simulink model "surgicalControl_Shared_memory_loop_2016a"  (R2016a)
settings: Solver=FixedStepAuto  SolverMode=SingleTasking  StartTime=0.0  StopTime=inf  FixedStep=1/100  RelTol=1e-3
libraries: dspsigops x9, simulink x3, matlabGenericSHM_Block x2
settings Model: Creator=daniel  LastModifiedBy=Bogdan
settings DebuggingCC: SFUnexpectedBacktrackingDiag=error  SFNoUnconditionalDefaultTransitionDiag=error
settings GRTTargetCC: TargetLangStandard=C99 (ISO)  GeneratePreprocessorConditionals=Use local settings
settings ConfigComp: CovMetricSettings=dwe  CovHtmlReporting=off  CovSaveCumulativeToWorkspaceVar=off  CovSaveSingleToWorkspaceVar=off  CovExternalEMLEnable=on

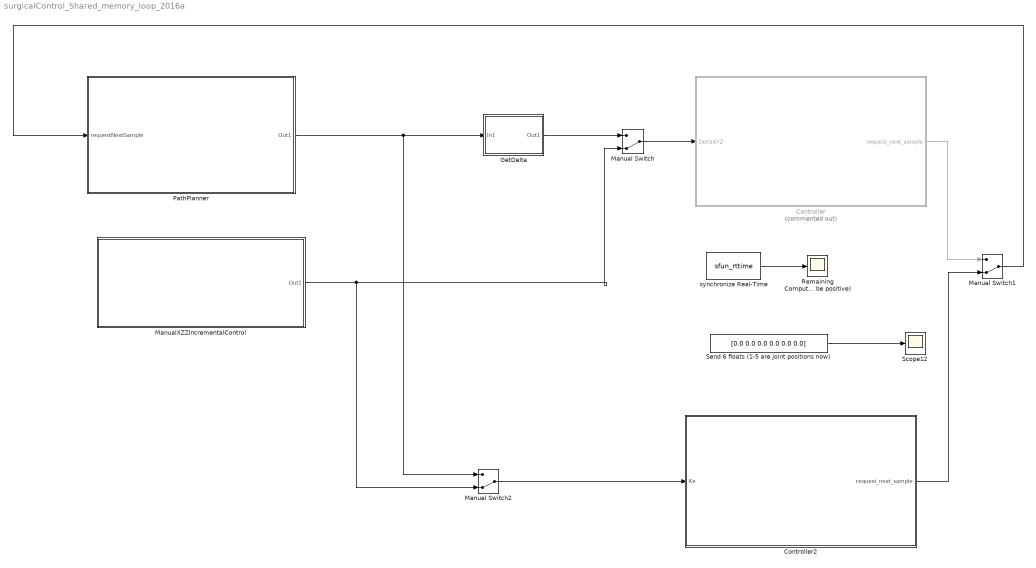
== system surgicalControl_Shared_memory_loop_2016a ==
  " GetDelta " : Subsystem
  Controller : Subsystem  Commented=on
  Controller2 : Subsystem
  Manual Switch : ManualSwitch  CurrentSetting=0
  Manual Switch1 : ManualSwitch  CurrentSetting=0
  Manual Switch2 : ManualSwitch  CurrentSetting=0
  "ManualXZZIncrementalControl " : Subsystem
  PathPlanner : Subsystem
  Remaining Computation Time (must be positive) : Scope
  Scope12 : Scope
  Send 6 floats (1-5 are joint positions now) : Constant  Value=[0.0 0.0 0.0 0.0 0.0 0.0]  OutDataTypeStr=single
  synchronize Real-Time : S-Function  FunctionName=sfun_rttime  Parameters=1  SFunctionDeploymentMode=off  EnableBusSupport=off
  wires:
  synchronize Real-Time/1 -> Remaining Computation Time (must be positive)/1
  Send 6 floats (1-5 are joint positions now)/1 -> Scope12/1
  "ManualXZZIncrementalControl "/1(Out1) -> Manual Switch2/2, Manual Switch/2
  " GetDelta "/1(Out1) -> Manual Switch/1
  Controller/1(request_next_sample) -> Manual Switch1/1
  Manual Switch/1 -> Controller/1(DeltaXYZ)
  PathPlanner/1(Out1) -> Manual Switch2/1, " GetDelta "/1(In1)
  Controller2/1(request_next_sample) -> Manual Switch1/2
  Manual Switch1/1 -> PathPlanner/1(requestNextSample)
  Manual Switch2/1 -> Controller2/1(Ke)

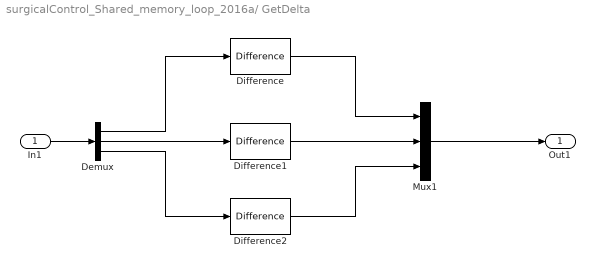
== system surgicalControl_Shared_memory_loop_2016a/ GetDelta  ==
  In1 : Inport
  Demux : Demux  Outputs=3
  Difference : simulink/Discrete/Difference  ICPrevInput=0  OutMin=[]  OutMax=[]  OutDataType=fixdt(1, 16)  OutScaling=2^-10  DoSatur=off
  Difference1 : simulink/Discrete/Difference  ICPrevInput=0  OutMin=[]  OutMax=[]  OutDataType=fixdt(1, 16)  OutScaling=2^-10  DoSatur=off
  Difference2 : simulink/Discrete/Difference  ICPrevInput=0  OutMin=[]  OutMax=[]  OutDataType=fixdt(1, 16)  OutScaling=2^-10  DoSatur=off
  Mux1 : Mux  Inputs=3
  Out1 : Outport
  wires:
  In1/1 -> Demux/1
  Demux/1 -> Difference/1
  Demux/2 -> Difference1/1
  Demux/3 -> Difference2/1
  Difference1/1 -> Mux1/2
  Difference/1 -> Mux1/1
  Difference2/1 -> Mux1/3
  Mux1/1 -> Out1/1

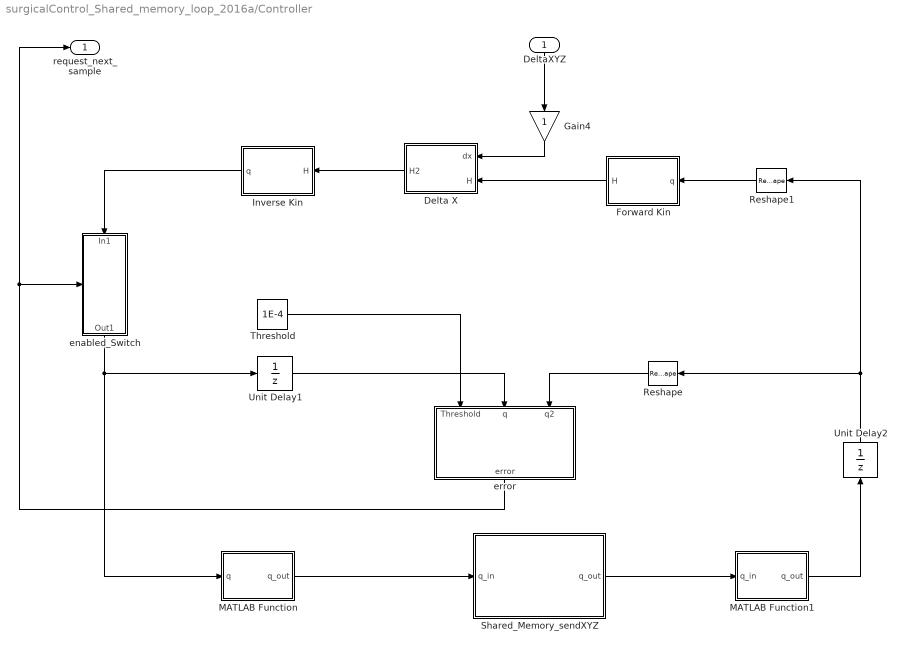
== system surgicalControl_Shared_memory_loop_2016a/Controller ==
  DeltaXYZ : Inport
  Delta X : MATLAB Function  TreatAsAtomicUnit=on
      settings: PermitHierarchicalResolution=ParametersOnly
  Forward Kin : MATLAB Function  TreatAsAtomicUnit=on
      settings: PermitHierarchicalResolution=ParametersOnly
  Gain4 : Gain
  Inverse Kin : MATLAB Function  TreatAsAtomicUnit=on
      settings: PermitHierarchicalResolution=ParametersOnly
  MATLAB Function : MATLAB Function  TreatAsAtomicUnit=on
      settings: PermitHierarchicalResolution=ParametersOnly
  MATLAB Function1 : MATLAB Function  TreatAsAtomicUnit=on
      settings: PermitHierarchicalResolution=ParametersOnly
  Reshape : Reshape
  Reshape1 : Reshape  OutputDimensionality=Customize  OutputDimensions=[1,6]
  Shared_Memory_sendXYZ : Subsystem  mask{ID1=4}
  "Threshold " : Constant  Value=1E-4
  Unit Delay1 : UnitDelay  InitialCondition=[0.0 0.0 0.0 0.0 0.0 0.0]  SampleTime=-1
  Unit Delay2 : UnitDelay  InitialCondition=[0.0 0.0 0.0 0.0 0.0 0.0]  SampleTime=-1
  "enabled_Switch " : Subsystem  TreatAsAtomicUnit=on
  error : MATLAB Function  TreatAsAtomicUnit=on
      settings: PermitHierarchicalResolution=ParametersOnly
  request_next_sample : Outport
  wires:
  Reshape/1 -> error/3(q2)
  MATLAB Function1/1(q_out) -> Unit Delay2/1
  Shared_Memory_sendXYZ/1(q_out) -> MATLAB Function1/1(q_in)
  Gain4/1 -> Delta X/1(dx)
  Forward Kin/1(H) -> Delta X/2(H)
  DeltaXYZ/1 -> Gain4/1
  Reshape1/1 -> Forward Kin/1(q)
  Unit Delay2/1 -> Reshape/1, Reshape1/1
  "enabled_Switch "/1(Out1) -> Unit Delay1/1, MATLAB Function/1(q)
  MATLAB Function/1(q_out) -> Shared_Memory_sendXYZ/1(q_in)
  error/1(error) -> request_next_sample/1, "enabled_Switch "/Enable
  Unit Delay1/1 -> error/2(q)
  Delta X/1(H2) -> Inverse Kin/1(H)
  Inverse Kin/1(q) -> "enabled_Switch "/1(In1)
  "Threshold "/1 -> error/1(Threshold)

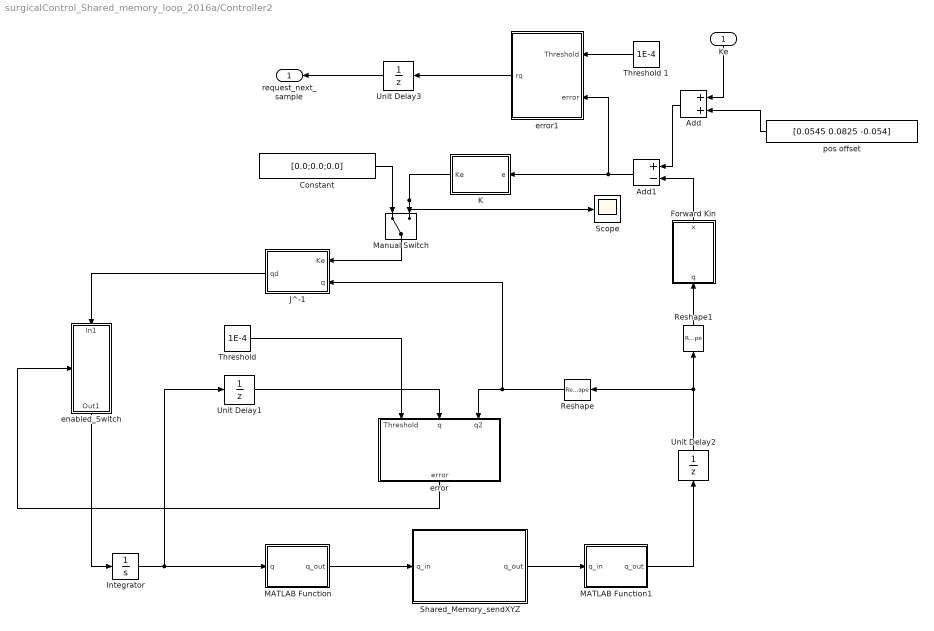
== system surgicalControl_Shared_memory_loop_2016a/Controller2 ==
  Ke : Inport
  Add : Sum
  Add1 : Sum  Inputs=+-
  Constant : Constant  Value=[0.0;0.0;0.0]
  Forward Kin : MATLAB Function  TreatAsAtomicUnit=on
      settings: PermitHierarchicalResolution=ParametersOnly
  Integrator : Integrator
  J^-1 : MATLAB Function  TreatAsAtomicUnit=on
      settings: PermitHierarchicalResolution=ParametersOnly
  K : Subsystem
  MATLAB Function : MATLAB Function  TreatAsAtomicUnit=on
      settings: PermitHierarchicalResolution=ParametersOnly
  MATLAB Function1 : MATLAB Function  TreatAsAtomicUnit=on
      settings: PermitHierarchicalResolution=ParametersOnly
  Manual Switch : ManualSwitch
  Reshape : Reshape
  Reshape1 : Reshape  OutputDimensionality=Customize  OutputDimensions=[1,6]
  Scope : Scope
  Shared_Memory_sendXYZ : Subsystem  mask{ID1=4}
  "Threshold " : Constant  Value=1E-4
  Threshold 1 : Constant  Value=1E-4
  Unit Delay1 : UnitDelay  InitialCondition=[0.0 0.0 0.0 0.0 0.0 0.0]  SampleTime=-1
  Unit Delay2 : UnitDelay  InitialCondition=[0.0 0.0 0.0 0.0 0.0 0.0]  SampleTime=-1
  Unit Delay3 : UnitDelay  SampleTime=-1
  "enabled_Switch " : Subsystem  TreatAsAtomicUnit=on
  error : MATLAB Function  TreatAsAtomicUnit=on
      settings: PermitHierarchicalResolution=ParametersOnly
  error1 : MATLAB Function  TreatAsAtomicUnit=on
      settings: PermitHierarchicalResolution=ParametersOnly
  "pos offset " : Constant  Value=[0.0545 0.0825 -0.054]  OutDataTypeStr=single
  request_next_sample : Outport
  wires:
  "Threshold "/1 -> error/1(Threshold)
  Unit Delay1/1 -> error/2(q)
  error/1(error) -> "enabled_Switch "/Enable
  Unit Delay2/1 -> Reshape1/1, Reshape/1
  Reshape1/1 -> Forward Kin/1(q)
  Shared_Memory_sendXYZ/1(q_out) -> MATLAB Function1/1(q_in)
  MATLAB Function1/1(q_out) -> Unit Delay2/1
  Reshape/1 -> J^-1/2(q), error/3(q2)
  J^-1/1(qd) -> "enabled_Switch "/1(In1)
  Integrator/1 -> MATLAB Function/1(q), Unit Delay1/1
  MATLAB Function/1(q_out) -> Shared_Memory_sendXYZ/1(q_in)
  Manual Switch/1 -> J^-1/1(Ke)
  Constant/1 -> Manual Switch/1
  Ke/1 -> Add/1
  Add1/1 -> error1/2(error), K/1(e)
  Add/1 -> Add1/1
  "pos offset "/1 -> Add/2
  Forward Kin/1(x) -> Add1/2
  K/1(Ke) -> Scope/1, Manual Switch/2
  "enabled_Switch "/1(Out1) -> Integrator/1
  Threshold 1/1 -> error1/1(Threshold)
  Unit Delay3/1 -> request_next_sample/1
  error1/1(rq) -> Unit Delay3/1

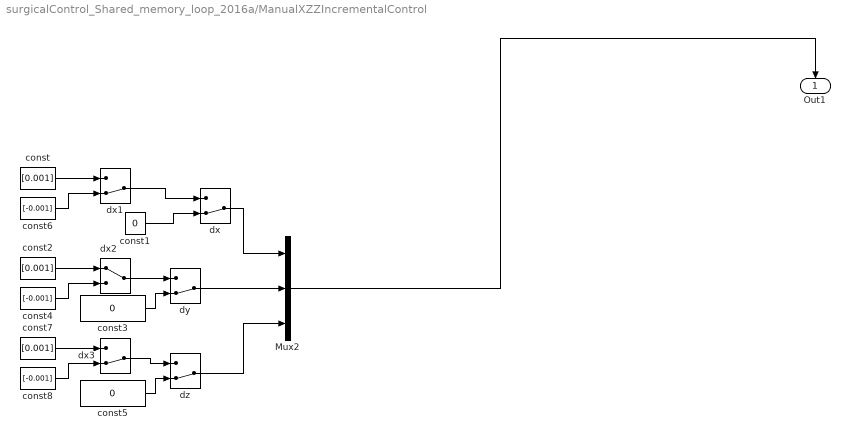
== system surgicalControl_Shared_memory_loop_2016a/ManualXZZIncrementalControl  ==
  Mux2 : Mux  Inputs=3
  const : Constant  Value=[0.001]  OutDataTypeStr=single
  const1 : Constant  Value=0  OutDataTypeStr=single
  const2 : Constant  Value=[0.001]  OutDataTypeStr=single
  const3 : Constant  Value=0  OutDataTypeStr=single
  const4 : Constant  Value=[-0.001]  OutDataTypeStr=single
  const5 : Constant  Value=0  OutDataTypeStr=single
  const6 : Constant  Value=[-0.001]  OutDataTypeStr=single
  const7 : Constant  Value=[0.001]  OutDataTypeStr=single
  const8 : Constant  Value=[-0.001]  OutDataTypeStr=single
  dx : ManualSwitch  CurrentSetting=0
  dx1 : ManualSwitch  CurrentSetting=0
  dx2 : ManualSwitch
  dx3 : ManualSwitch  CurrentSetting=0
  dy : ManualSwitch  CurrentSetting=0
  dz : ManualSwitch  CurrentSetting=0
  Out1 : Outport
  wires:
  const/1 -> dx1/1
  const6/1 -> dx1/2
  const2/1 -> dx2/1
  dz/1 -> Mux2/3
  dx/1 -> Mux2/1
  dx2/1 -> dy/1
  dy/1 -> Mux2/2
  dx3/1 -> dz/1
  const5/1 -> dz/2
  Mux2/1 -> Out1/1
  const8/1 -> dx3/2
  const7/1 -> dx3/1
  const3/1 -> dy/2
  const1/1 -> dx/2
  dx1/1 -> dx/1
  const4/1 -> dx2/2

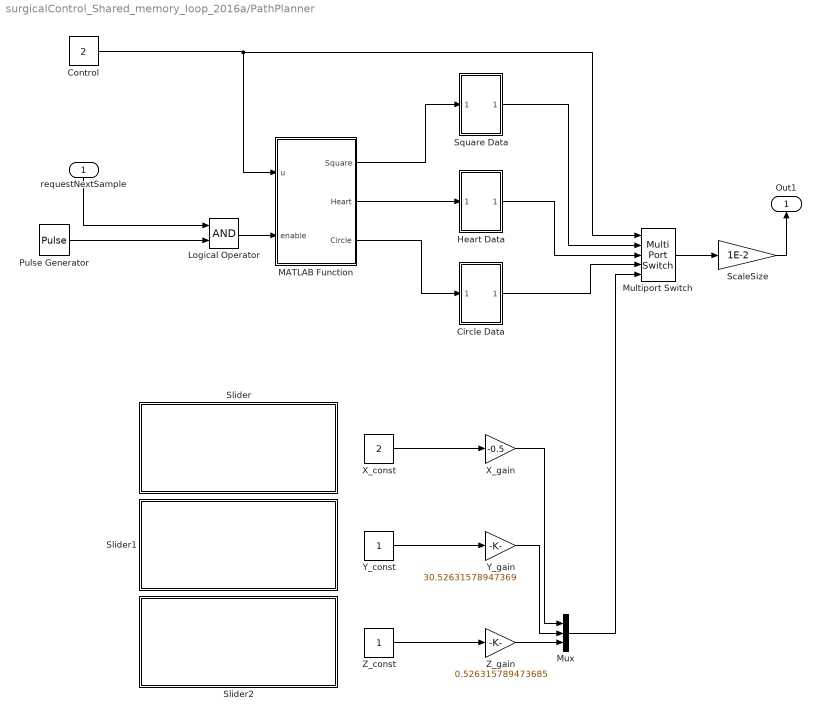
== system surgicalControl_Shared_memory_loop_2016a/PathPlanner ==
  requestNextSample : Inport
  " X_const " : Constant  Value=2
  " Y_const" : Constant
  " Z_const" : Constant
  Circle Data : Subsystem
  "Control " : Constant  Value=2
  Heart Data : Subsystem
  Logical Operator : Logic  AllPortsSameDT=off  OutDataTypeStr=boolean
  MATLAB Function : MATLAB Function  TreatAsAtomicUnit=on
      settings: PermitHierarchicalResolution=ParametersOnly
  Multiport Switch : MultiPortSwitch  Inputs=4
  Mux : Mux  Inputs=3
  Pulse Generator : DiscretePulseGenerator  PulseType=Time based  Period=0.1  PulseWidth=50
  ScaleSize : Gain  Gain=1E-2
  Slider : Subsystem  DialogController=hmiCreateDDGDialog  IsWebBlock=on  mask(MWDashboardBlock){webBlockId=4f94596f-dd6d-4e5e-bddc-7a8d913927f9, webBlockType=slider, ShowInLibBrowser=on, ShowInitialText=on, HMISrcModelName=surgicalControl_Shared_memory_loop_2016a}
      mask prompts: webBlockId "WebBlock Id"; webBlockType "WebBlock Type"; HMISrcModelName "Source Model"
      mask help: SimulinkHMI:dialogs:SliderDialogDesc
      mask Help: helpview([docroot '/mapfiles/simulink.map'], 'hmi_slider')
      mask Display:
      | if strcmp(get_param(bdroot(gcb),'BlockDiagramType'), 'library')
      |     image([(matlabroot) '/toolbox/simulink/hmi/icons/Slider.png']);
      | end
  Slider1 : Subsystem  DialogController=hmiCreateDDGDialog  IsWebBlock=on  mask(MWDashboardBlock){webBlockId=8aa996ad-7cd4-40fc-9a04-6a85939aea5d, webBlockType=slider, ShowInLibBrowser=on, ShowInitialText=on, HMISrcModelName=surgicalControl_Shared_memory_loop_2016a}
      mask prompts: webBlockId "WebBlock Id"; webBlockType "WebBlock Type"; HMISrcModelName "Source Model"
      mask help: SimulinkHMI:dialogs:SliderDialogDesc
      mask Help: helpview([docroot '/mapfiles/simulink.map'], 'hmi_slider')
      mask Display:
      | if strcmp(get_param(bdroot(gcb),'BlockDiagramType'), 'library')
      |     image([(matlabroot) '/toolbox/simulink/hmi/icons/Slider.png']);
      | end
  Slider2 : Subsystem  DialogController=hmiCreateDDGDialog  IsWebBlock=on  mask(MWDashboardBlock){webBlockId=1ddf6fd9-0225-4881-82ca-a25e179e2ab9, webBlockType=slider, ShowInLibBrowser=on, ShowInitialText=on, HMISrcModelName=surgicalControl_Shared_memory_loop_2016a}
      mask prompts: webBlockId "WebBlock Id"; webBlockType "WebBlock Type"; HMISrcModelName "Source Model"
      mask help: SimulinkHMI:dialogs:SliderDialogDesc
      mask Help: helpview([docroot '/mapfiles/simulink.map'], 'hmi_slider')
      mask Display:
      | if strcmp(get_param(bdroot(gcb),'BlockDiagramType'), 'library')
      |     image([(matlabroot) '/toolbox/simulink/hmi/icons/Slider.png']);
      | end
  "Square Data " : Subsystem
  "X_gain " : Gain  Gain=-0.5
  "Y_gain " : Gain  Gain=30.52631578947369
  Z_gain : Gain  Gain=0.526315789473685
  Out1 : Outport
  wires:
  " Z_const"/1 -> Z_gain/1
  Z_gain/1 -> Mux/3
  "X_gain "/1 -> Mux/1
  "Control "/1 -> MATLAB Function/1(u), Multiport Switch/1
  Multiport Switch/1 -> ScaleSize/1
  " X_const "/1 -> "X_gain "/1
  ScaleSize/1 -> Out1/1
  " Y_const"/1 -> "Y_gain "/1
  "Y_gain "/1 -> Mux/2
  Pulse Generator/1 -> Logical Operator/2
  requestNextSample/1 -> Logical Operator/1
  MATLAB Function/1(Square) -> "Square Data "/1(In1)
  Logical Operator/1 -> MATLAB Function/2(enable)
  MATLAB Function/2(Heart) -> Heart Data/1(In1)
  MATLAB Function/3(Circle) -> Circle Data/1(In1)
  "Square Data "/1(xyz) -> Multiport Switch/2
  Heart Data/1(xyz) -> Multiport Switch/3
  Circle Data/1(xyz) -> Multiport Switch/4
  Mux/1 -> Multiport Switch/5

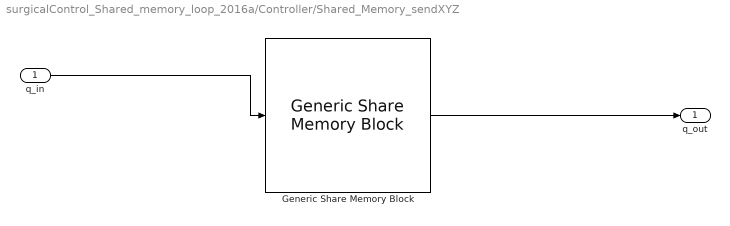
== system surgicalControl_Shared_memory_loop_2016a/Controller/Shared_Memory_sendXYZ ==
  q_in : Inport
  Generic Share Memory Block : matlabGenericSHM_Block/Generic Share Memory Block  nombre='EyeRob'  dispositivo=ID1  vecE=[6]  vecS=[6]  tipoE=['f']  tipoS=['f']
  q_out : Outport
  wires:
  q_in/1 -> Generic Share Memory Block/1
  Generic Share Memory Block/1 -> q_out/1

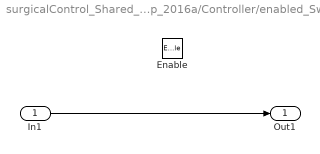
== system surgicalControl_Shared_memory_loop_2016a/Controller/enabled_Switch  ==
  In1 : Inport
  Enable : EnablePort
  Out1 : Outport
  wires:
  In1/1 -> Out1/1

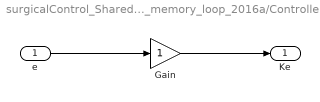
== system surgicalControl_Shared_memory_loop_2016a/Controller2/K ==
  e : Inport
  Gain : Gain
  Ke : Outport
  wires:
  Gain/1 -> Ke/1
  e/1 -> Gain/1

== system surgicalControl_Shared_memory_loop_2016a/Controller2/Shared_Memory_sendXYZ ==
  q_in : Inport
  Generic Share Memory Block : matlabGenericSHM_Block/Generic Share Memory Block  nombre='EyeRob'  dispositivo=ID1  vecE=[6]  vecS=[6]  tipoE=['f']  tipoS=['f']
  q_out : Outport
  wires:
  Generic Share Memory Block/1 -> q_out/1
  q_in/1 -> Generic Share Memory Block/1

== system surgicalControl_Shared_memory_loop_2016a/Controller2/enabled_Switch  ==
  In1 : Inport
  Enable : EnablePort
  Out1 : Outport
  wires:
  In1/1 -> Out1/1

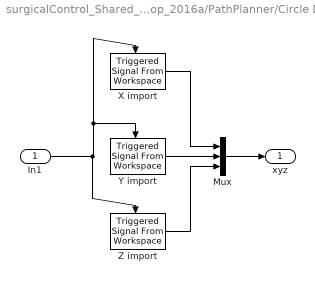
== system surgicalControl_Shared_memory_loop_2016a/PathPlanner/Circle Data ==
  In1 : Inport
  Mux : Mux  Inputs=3
  X import : dspsigops/Triggered Signal From Workspace  Signal=xs_circle  TriggerType=Falling edge  ic=0  SamplesPerFrame=1  OutputAfterFinalValue=Setting to zero  OutputFrames=off
  Y import : dspsigops/Triggered Signal From Workspace  Signal=ys_circle  TriggerType=Falling edge  ic=0  SamplesPerFrame=1  OutputAfterFinalValue=Setting to zero  OutputFrames=off
  Z import : dspsigops/Triggered Signal From Workspace  Signal=zs_circle  TriggerType=Falling edge  ic=0  SamplesPerFrame=1  OutputAfterFinalValue=Setting to zero  OutputFrames=off
  xyz : Outport
  wires:
  X import/1 -> Mux/1
  Z import/1 -> Mux/3
  Mux/1 -> xyz/1
  Y import/1 -> Mux/2
  In1/1 -> Z import/Trigger, X import/Trigger, Y import/Trigger

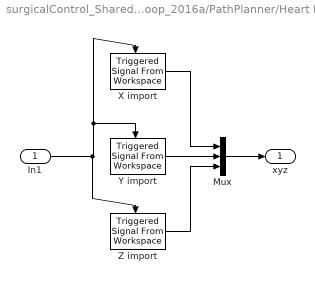
== system surgicalControl_Shared_memory_loop_2016a/PathPlanner/Heart Data ==
  In1 : Inport
  Mux : Mux  Inputs=3
  X import : dspsigops/Triggered Signal From Workspace  Signal=xs_heart  TriggerType=Falling edge  ic=0  SamplesPerFrame=1  OutputAfterFinalValue=Setting to zero  OutputFrames=off
  Y import : dspsigops/Triggered Signal From Workspace  Signal=ys_heart  TriggerType=Falling edge  ic=0  SamplesPerFrame=1  OutputAfterFinalValue=Setting to zero  OutputFrames=off
  Z import : dspsigops/Triggered Signal From Workspace  Signal=zs_heart  TriggerType=Falling edge  ic=0  SamplesPerFrame=1  OutputAfterFinalValue=Setting to zero  OutputFrames=off
  xyz : Outport
  wires:
  X import/1 -> Mux/1
  Z import/1 -> Mux/3
  Mux/1 -> xyz/1
  Y import/1 -> Mux/2
  In1/1 -> Z import/Trigger, X import/Trigger, Y import/Trigger

== system surgicalControl_Shared_memory_loop_2016a/PathPlanner/Slider ==

== system surgicalControl_Shared_memory_loop_2016a/PathPlanner/Slider1 ==

== system surgicalControl_Shared_memory_loop_2016a/PathPlanner/Slider2 ==

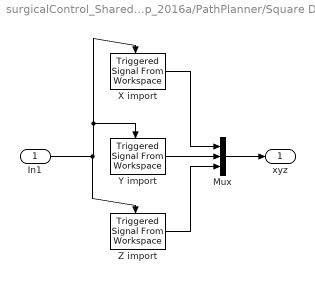
== system surgicalControl_Shared_memory_loop_2016a/PathPlanner/Square Data  ==
  In1 : Inport
  Mux : Mux  Inputs=3
  X import : dspsigops/Triggered Signal From Workspace  Signal=xs_square  TriggerType=Falling edge  ic=0  SamplesPerFrame=1  OutputAfterFinalValue=Setting to zero  OutputFrames=off
  Y import : dspsigops/Triggered Signal From Workspace  Signal=ys_square  TriggerType=Falling edge  ic=0  SamplesPerFrame=1  OutputAfterFinalValue=Setting to zero  OutputFrames=off
  Z import : dspsigops/Triggered Signal From Workspace  Signal=zs_square  TriggerType=Falling edge  ic=0  SamplesPerFrame=1  OutputAfterFinalValue=Setting to zero  OutputFrames=off
  xyz : Outport
  wires:
  X import/1 -> Mux/1
  Z import/1 -> Mux/3
  Mux/1 -> xyz/1
  Y import/1 -> Mux/2
  In1/1 -> Z import/Trigger, X import/Trigger, Y import/Trigger

== matlab function surgicalControl_Shared_memory_loop_2016a/PathPlanner/MATLAB Function ==
  data: u input; Square output; enable input; Heart output; Circle output
function [Square,Heart,Circle] = fcn(u,enable)
%#codegen

Square = enable && (u==1);
Heart = enable && (u==2);
Circle = enable && (u==3);

== matlab function surgicalControl_Shared_memory_loop_2016a/Controller/Forward Kin ==
  data: q input; H output
function H = fcn(q)
H = fKin(q);

== matlab function surgicalControl_Shared_memory_loop_2016a/Controller2/J^-1 ==
  data: Ke input; q input; qd output
function qd = fcn(Ke,q)
qd = j_Tool(q',0)*[Ke;0;0];

== matlab function surgicalControl_Shared_memory_loop_2016a/Controller/error ==
  data: Threshold input; q input; error output; q2 input
function error = fcn(Threshold,q,q2)
H1 = fKin(q');
H2 = fKin(q2');
H=H1-H2;
error=(norm(H(1:3,4)')<Threshold);
end

== matlab function surgicalControl_Shared_memory_loop_2016a/Controller/MATLAB Function ==
  data: q input size=[1 6]; q_out output size=[1 6]
function q_out = correctForPrismatic(q)
%#codegen
 if iscolumn(q)
       q = q';
 end
q_out=zeros(1, 6,'single');
offsetX=0.00489158;
offsetY=-0.000502541;
q1=q(1,1);
q2=q(1,2);
q3=q(1,3);
q4=q(1,4);
q2_temp= getL2(q1,q2);
q4_temp= getL1(q3,q4);

% end


q_out(1,1) = q1+offsetX;
q_out(1,2) = q2_temp;
q_out(1,3) = q3+offsetY;
q_out(1,4) = q4_temp;
q_out(1,5) = q(1,5);
q_out(1,6) = q(1,6);
end

== matlab function surgicalControl_Shared_memory_loop_2016a/Controller/MATLAB Function1 ==
  data: q_in input size=[1 6]; q_out output size=[1 6]
function q_out = recorrectForPrismatic(q_in)
%#codegen
q=q_in;
q_out=zeros(1, 6,'double');
d= 17e-3;
offsetX=0.00489158;
offsetY=-0.000502541;

q1=q(1,1)-offsetX;
q2=q(1,2);
q3=q(1,3)-offsetY;
q4=q(1,4);
q2_temp= atan((q2-q1)/d);
q4_temp= atan((q3-q4)/d); 

% end
%q_out=[q1,q2_temp,q3,q4_temp,q(1,5),q(1,6)];

q_out(1,1) = q1;
q_out(1,2) = q2_temp;
q_out(1,3) = q3;
q_out(1,4) = q4_temp;
q_out(1,5) = q(1,5);
q_out(1,6) = q(1,6);
%q_out=round(q_out*1000)/1000;
end

== matlab function surgicalControl_Shared_memory_loop_2016a/Controller/Inverse Kin ==
  data: H input; q output
function q = fcn(H)

%q = round(IK(H)'*1000)/1000;
q = IK(H)';

== matlab function surgicalControl_Shared_memory_loop_2016a/Controller/Delta X ==
  data: dx input; H input; H2 output
function H2 = fcn(dx,H)
H2 = H;
H2(1,4)=H2(1,4)+dx(3,1);
H2(2,4)=H2(2,4)+dx(2,1);
H2(3,4)=H2(3,4)+dx(1,1);
end

== matlab function surgicalControl_Shared_memory_loop_2016a/Controller2/Forward Kin ==
  data: q input; x output
function x = fcn(q)
H = fKin(q);
x=H(3:-1:1,4);

== matlab function surgicalControl_Shared_memory_loop_2016a/Controller2/error1 ==
  data: Threshold input; error input; rq output
function rq = fcn(Threshold,error)
rq=(norm(error)<Threshold);
end

== matlab function surgicalControl_Shared_memory_loop_2016a/Controller2/MATLAB Function ==
  data: q input size=[1 6]; q_out output size=[1 6]
function q_out = correctForPrismatic(q)
%#codegen
 if iscolumn(q)
       q = q';
 end
q_out=zeros(1, 6,'single');
offsetX=0.00489158;
offsetY=-0.000502541;
q1=q(1,1);
q2=q(1,2);
q3=q(1,3);
q4=q(1,4);
q2_temp= getL2(q1,q2);
q4_temp= getL1(q3,q4);

% end


q_out(1,1) = q1+offsetX;
q_out(1,2) = q2_temp;
q_out(1,3) = q3+offsetY;
q_out(1,4) = q4_temp;
q_out(1,5) = q(1,5);
q_out(1,6) = q(1,6);
end

== matlab function surgicalControl_Shared_memory_loop_2016a/Controller2/MATLAB Function1 ==
  data: q_in input size=[1 6]; q_out output size=[1 6]
function q_out = recorrectForPrismatic(q_in)
%#codegen
q=q_in;
q_out=zeros(1, 6,'double');
d= 17e-3;
offsetX=0.00489158;
offsetY=-0.000502541;

q1=q(1,1)-offsetX;
q2=q(1,2);
q3=q(1,3)-offsetY;
q4=q(1,4);
q2_temp= atan((q2-q1)/d);
q4_temp= atan((q3-q4)/d); 

% end
%q_out=[q1,q2_temp,q3,q4_temp,q(1,5),q(1,6)];

q_out(1,1) = q1;
q_out(1,2) = q2_temp;
q_out(1,3) = q3;
q_out(1,4) = q4_temp;
q_out(1,5) = q(1,5);
q_out(1,6) = q(1,6);
%q_out=round(q_out*1000)/1000;
end

== matlab function surgicalControl_Shared_memory_loop_2016a/Controller2/error ==
  data: Threshold input; q input; error output; q2 input
function error = fcn(Threshold,q,q2)
H1 = fKin(q');
H2 = fKin(q2');
H=H1-H2;
error=(norm(H(1:3,4)')<Threshold);
end
